simulink model "PStest"  (R2018a)
settings: Solver=VariableStepAuto  StartTime=0.0  StopTime=5  RelTol=1e-8
PreLoadFcn:
  | Ts_Power=50e-6;
  | Ts_Control=100e-6;
StopFcn:
  | clear C
  | C(1,:)={'Iterac',saveIte(1,1),saveIte(1,2),saveIte(1,3),saveIte(1,4)};
  | C(2,:)={'Time (sec)',saveIte(2,1),saveIte(2,2),saveIte(2,3),saveIte(2,4)};
  | C(3,:)={'Pmax',saveIte(3,1),saveIte(3,2),saveIte(3,3),saveIte(3,4)};
  | C(4,:)={'Duty',saveIte(4,1),saveIte(4,2),saveIte(4,3),saveIte(4,4)};
  | C(5,:)={'When',saveIte(5,1)*0.1,saveIte(5,2)*0.1,saveIte(5,3)*0.1,saveIte(5,4)*0.1};
  | C(6,:)={'Tolerac',saveIte(6,1),saveIte(6,2),saveIte(6,3),saveIte(6,4)};
  | openvar('C')
libraries: powerlib x19, re_lib x6, simulink x1
Description:
  | Copyright 2008-2018 The MathWorks, Inc.
settings Model: NumberOfSteps=8002  Creator=MathWorks  LastModifiedBy=Mortuus
settings DataIOCC: LimitDataPoints=on  SaveFormat=Array  SignalLoggingSaveFormat=ModelDataLogs
settings OptimizationCC: ExpressionDepthLimit=2147483647  LifeSpan=inf
settings DebuggingCC: AlgebraicLoopMsg=none  UnderspecifiedInitializationDetection=Classic  MergeDetectMultiDrivingBlocksExec=none  SolverPrmCheckMsg=warning  FcnCallInpInsideContextMsg=warning  StateNameClashWarn=warning  SFUnexpectedBacktrackingDiag=warning  SFNoUnconditionalDefaultTransitionDiag=warning  SFExecutionAtInitializationDiag=none
settings HardwareCC: ProdBitPerPointer=32  ProdBitPerSizeT=32  ProdBitPerPtrDiffT=32  ProdLargestAtomicFloat=None  ProdIntDivRoundTo=Undefined  ProdEndianess=Unspecified  ProdWordSize=32  ProdHWDeviceType=32-bit Generic
settings ModelReferenceCC: PropagateSignalLabelsOutOfModel=off
settings CodeAppCC: StateflowObjectComments=on
settings GRTTargetCC: TargetLangStandard=C89/C90 (ANSI)  GeneratePreprocessorConditionals=Disable all  CombineOutputUpdateFcns=off  GRTInterface=on
settings ConfigComp: CovMetricSettings=dw  CovHtmlReporting=on  CovSaveCumulativeToWorkspaceVar=on  CovSaveSingleToWorkspaceVar=on  CovExternalEMLEnable=off  CovSFcnEnable=off
settings SimscapeCC: SimscapeNormalizeSystem=off

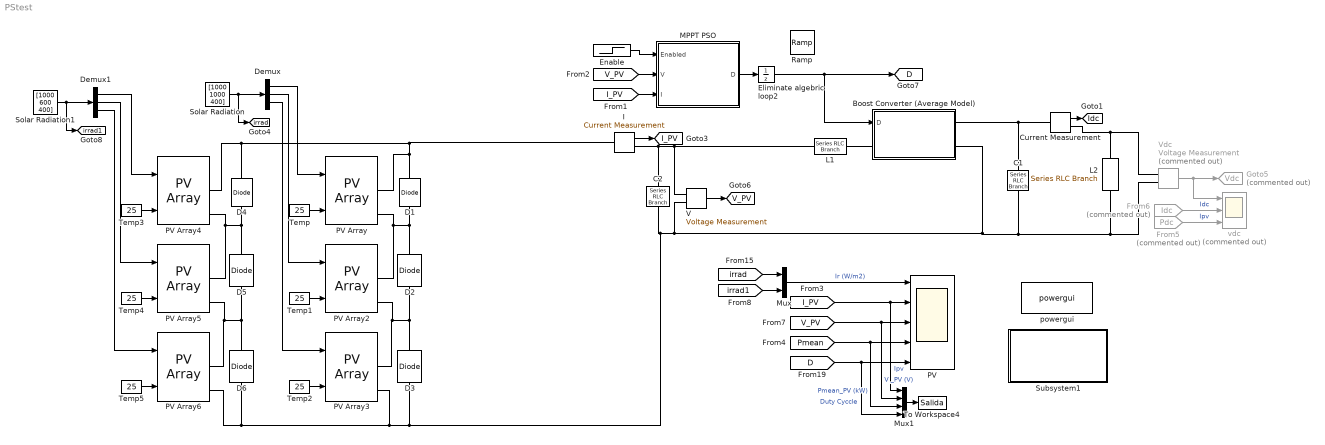
== system PStest ==
  Boost Converter (Average Model) : Subsystem  mask(Boost Converter (Average Model)){Ts=Ts_Power}
      mask prompts: Ts "Sample time:"
      mask Display: disp('Boost\n(Average)')
  C1 : powerlib/Elements/Series RLC Branch  LConnTagsString=__new0  RConnTagsString=__new0  BranchType=C  Resistance=1.0  Inductance=1.0  SetiL0=off  InitialCurrent=0  Capacitance=220e-06  Setx0=on  InitialVoltage=1  Measurements=None
  C2 : powerlib/Elements/Series RLC Branch  LConnTagsString=__new0  RConnTagsString=__new0  BranchType=C  Resistance=1.0  Inductance=1.0  SetiL0=off  InitialCurrent=0  Capacitance=470e-6  Setx0=on  InitialVoltage=50  Measurements=Branch voltage
  Current Measurement : powerlib/Measurements/Current Measurement  PhasorSimulation=off  OutputType=Magnitude  PSBequivalent=0
  D{1..6} (6 alike) : powerlib/Power Electronics/Diode  Ron=0.001  Lon=0  Vf=0.8  IC=0  UseSnubber=off  Rs=500  Cs=250e-9  Measurements=off
  Demux : Demux  Outputs=3
  Demux1 : Demux  Outputs=3
  Eliminate algebric loop2 : UnitDelay  SampleTime=Ts_Control
  Enable : Step  Time=0.01  SampleTime=0
  From5 : From  Commented=on  GotoTag=Pdc  TagVisibility=global
      settings: CloseFcn=tagdialog Close
  From6 : From  Commented=on  GotoTag=Idc  TagVisibility=global
      settings: CloseFcn=tagdialog Close
  Goto5 : Goto  Commented=on  GotoTag=Vdc  TagVisibility=global
  I : powerlib/Measurements/Current Measurement  PhasorSimulation=off  OutputType=Complex  PSBequivalent=0
  L1 : powerlib/Elements/Series RLC Branch  LConnTagsString=__new0  RConnTagsString=__new0  BranchType=RL  Resistance=0.3  Inductance=1e-3  SetiL0=off  InitialCurrent=0  Capacitance=1e-6  Setx0=off  InitialVoltage=0  Measurements=None
  L2 : powerlib/Elements/Series RLC Branch  LConnTagsString=__new0  RConnTagsString=__new0  BranchType=R  Resistance=100  Inductance=5e-3  SetiL0=off  InitialCurrent=0  Capacitance=1e-6  Setx0=off  InitialVoltage=0  Measurements=None
  "MPPT PSO " : MATLAB Function  TreatAsAtomicUnit=on  SystemSampleTime=0.1
  Mux : Mux  Inputs=2
  Mux1 : Mux
  PV : Scope  NumInputPorts=5
  PV Array{,2..6} (6 alike) : re_lib/Solar/PV Array  Npar=1  Nser=1  PlotType=array @ 25 deg.C & specified irradiances  S_vec="[ 1000  250 ]"  Temp_C_vec=[ 0 25 50]  ModuleName=User-defined  PlotWhenSelected=off  Pm=249.6159  Ncell=60  Voc=37.4  Isc=8.72  Vm=30.33  Im=8.23  beta_Voc_pc=-0.34  alpha_Isc_pc=0.07  beta_Voc=-0.12716  alpha_Isc=0.006104  IL=8.7463  I0=1.471e-10  nI=0.97837  Rsh=402.3586  Rs=0.31469  BAL=off  Tc=Tc  Tfilter=50e-6
  Ramp : simulink/Sources/Ramp  slope=-0.25  start=1  InitialOutput=1
  Solar Radiation : Constant  Value=[1000 1000 400]
  Solar Radiation1 : Constant  Value=[1000 600 400]
  Subsystem1 : Subsystem
      mask Display: disp('Additional \nscopes & measurements')
  Temp{,1..5} (6 alike) : Constant  Value=25
  To Workspace4 : ToWorkspace  VariableName=Salida  SaveFormat=Structure With Time  SampleTime=50e-6
      settings: Decimation=10
  V : powerlib/Measurements/Voltage Measurement  PhasorSimulation=off  OutputType=Complex  PSBequivalent=0
  "Vdc " : powerlib/Measurements/Voltage Measurement  Tag=PoWeRsYsTeMmEaSuReMeNt  Commented=on  PhasorSimulation=off  OutputType=Magnitude  PSBequivalent=0
  powergui : powerlib/powergui  Priority=1  SimulationMode=Continuous  SampleTime=Ts_Power  frequency=60  Iterations=50  frequencyindice=0  Pbase=100e6  ErrMax=1e-4  UnitsV=kV  UnitsW=MW  buscounter=0  FunctionMessages=off  echomessages=off  EnableUseOfTLC=off  CurrentSourceSwitches=off  DisableSnubberDevices=off  DisableRonSwitches=off  DisableVfSwitches=off  DisplayEquations=off  SolverType=Tustin/Backward Euler (TBE)  Interpol=off  ExternalGateDelay=off  methode=off  Ts=100  x0status=blocks  SPID=off  SwTol=0  HookPort=off  RestoreLinks=warning  ResistiveCurrentMeasurement=off  Frange=[0:2:500]  Ylog=off  Xlog=on  ShowGrid=off  save=off  variable=ZData  structure=0  ZoomFFT=on  StartTime=0.0  cycles=1  DisplayStyle=1  fundamental=60  FreqAxis=off  MaxFrequency=1000  frequencyindicesteady=1  RmsSteady=1  display=off
  vdc : Scope  Commented=on  NumInputPorts=3
  tag scope: D=global, I_PV=global, Idc=global, V_PV=global, irrad1=global, irrad=global
  wires:
  "MPPT PSO "/1(D) -> Eliminate algebric loop2/1
  [V_PV] -> "MPPT PSO "/2(V)
  [I_PV] -> "MPPT PSO "/3(I)
  Enable/1 -> "MPPT PSO "/1(Enabled)
  [Pmean] -> Mux1/3, PV/4  "Pmean_PV (kW)"
  [V_PV] -> Mux1/2, PV/3  "V _PV (V)"
  [I_PV] -> Mux1/1, PV/2  "Ipv"
  "Vdc "/1 -> vdc/1, Goto5/1
  Current Measurement/1 -> [Idc]
  From5/1 -> vdc/3  "Ipv"
  From6/1 -> vdc/2  "Idc"
  [D] -> Mux1/4, PV/5  "Duty Cyccle"
  I/1 -> [I_PV]
  V/1 -> [V_PV]
  Solar Radiation/1 -> [irrad], Demux/1
  Demux/1 -> PV Array/1
  Demux/2 -> PV Array2/1
  Demux/3 -> PV Array3/1
  Temp/1 -> PV Array/2
  Temp1/1 -> PV Array2/2
  Temp2/1 -> PV Array3/2
  Temp5/1 -> PV Array6/2
  Temp4/1 -> PV Array5/2
  Temp3/1 -> PV Array4/2
  Demux1/1 -> PV Array4/1
  Solar Radiation1/1 -> [irrad1], Demux1/1
  Demux1/3 -> PV Array6/1
  Demux1/2 -> PV Array5/1
  Eliminate algebric loop2/1 -> [D], Boost Converter (Average Model)/1(D)
  Mux/1 -> PV/1  "Ir (W/m2)"
  [irrad] -> Mux/1
  [irrad1] -> Mux/2
  Mux1/1 -> To Workspace4/1
  connections:
  L2/LConn1 -- Current Measurement/RConn1 -- "Vdc "/LConn1
  L1/RConn1 -- Boost Converter (Average Model)/LConn1
  Boost Converter (Average Model)/RConn1 -- Current Measurement/LConn1 -- C1/LConn1
  Boost Converter (Average Model)/RConn2 -- D6/LConn1 -- PV Array6/RConn2 -- PV Array3/RConn2 -- D3/LConn1 -- C2/RConn1 -- V/LConn2 -- C1/RConn1 -- L2/RConn1 -- "Vdc "/LConn2
  C2/LConn1 -- L1/LConn1 -- V/LConn1 -- I/RConn1
  D1/LConn1 -- D2/RConn1 -- PV Array2/RConn1 -- PV Array/RConn2
  D3/RConn1 -- PV Array2/RConn2 -- PV Array3/RConn1 -- D2/LConn1
  D1/RConn1 -- D4/RConn1 -- PV Array4/RConn1 -- I/LConn1 -- PV Array/RConn1
  PV Array6/RConn1 -- PV Array5/RConn2 -- D5/LConn1 -- D6/RConn1
  PV Array4/RConn2 -- PV Array5/RConn1 -- D5/RConn1 -- D4/LConn1

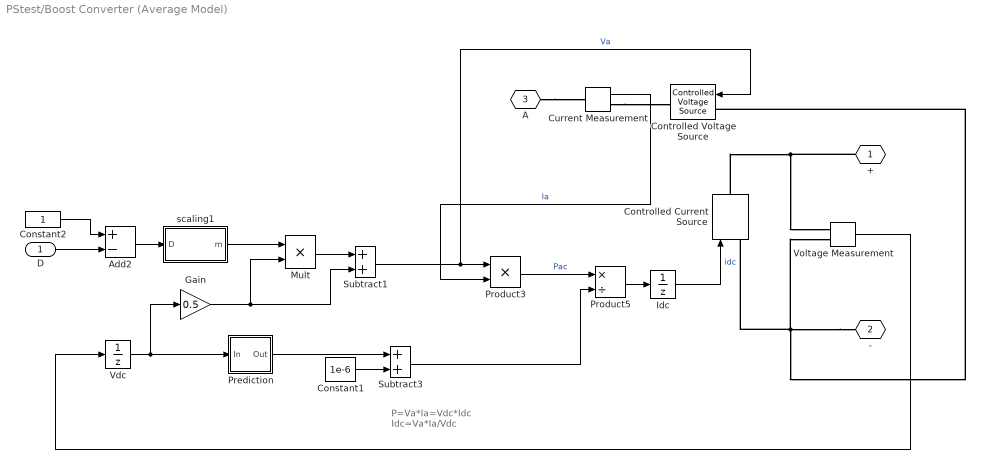
== system PStest/Boost Converter (Average Model) ==
  note: P=Va*Ia=Vdc*Idc
      | Idc=Va*Ia/Vdc
  D : Inport
  Add2 : Sum  Inputs=+-
  Constant1 : Constant  Value=1e-6
  Constant2 : Constant
  Controlled Current Source : powerlib/Electrical Sources/Controlled Current Source  Initialize=on  Source_Type=AC  Amplitude=0  Phase=0  Frequency=0  Measurements=None
  Controlled Voltage Source : powerlib/Electrical Sources/Controlled Voltage Source  Initialize=on  Source_Type=AC  Amplitude=0  Phase=0  Frequency=0  Measurements=None
  Current Measurement : powerlib/Measurements/Current Measurement  PhasorSimulation=off  OutputType=Complex  PSBequivalent=0
  Gain : Gain  Gain=0.5
  Idc : UnitDelay  SampleTime=Ts
  Mult : Product  Inputs=**
  Prediction : Subsystem
  Product3 : Product  RndMeth=Zero
  Product5 : Product  Inputs=*/  RndMeth=Zero
  Subtract1 : Sum
  Subtract3 : Sum
  Vdc : UnitDelay  SampleTime=Ts
  Voltage Measurement : powerlib/Measurements/Voltage Measurement  PhasorSimulation=off  OutputType=Complex  PSBequivalent=0
  scaling1 : Subsystem
  + : PMIOPort  Tag=PMCPort  Side=Right
  - : PMIOPort  Tag=PMCPort  Port=2  Side=Right
  A : PMIOPort  Tag=PMCPort  Port=3  Side=Left
  wires:
  Gain/1 -> Mult/2, Subtract1/2
  Product5/1 -> Idc/1
  Constant1/1 -> Subtract3/2
  Subtract3/1 -> Product5/2
  Product3/1 -> Product5/1  "Pac"
  Prediction/1(Out) -> Subtract3/1
  Vdc/1 -> Prediction/1(In), Gain/1
  Subtract1/1 -> Product3/1, Controlled Voltage Source/1  "Va"
  Mult/1 -> Subtract1/1
  Constant2/1 -> Add2/1
  Add2/1 -> scaling1/1(D)
  scaling1/1(m) -> Mult/1
  D/1 -> Add2/2
  Voltage Measurement/1 -> Vdc/1
  Idc/1 -> Controlled Current Source/1  "idc"
  Current Measurement/1 -> Product3/2  "Ia"
  connections:
  -/RConn1 -- Voltage Measurement/LConn2 -- Controlled Voltage Source/LConn1 -- Controlled Current Source/LConn1
  +/RConn1 -- Voltage Measurement/LConn1 -- Controlled Current Source/RConn1
  Current Measurement/RConn1 -- Controlled Voltage Source/RConn1
  A/RConn1 -- Current Measurement/LConn1

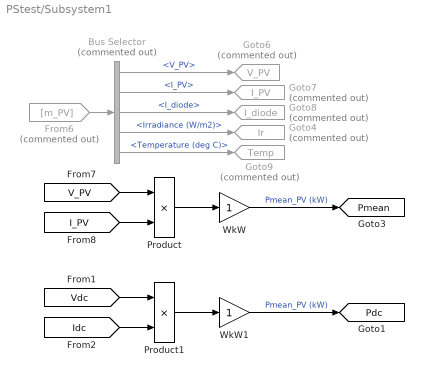
== system PStest/Subsystem1 ==
  Bus Selector : BusSelector  Commented=on  OutputSignals=V_PV,I_PV,I_diode,Irradiance (W/m2),Temperature (deg C)
  From6 : From  Commented=on  GotoTag=m_PV  TagVisibility=global
  Goto4 : Goto  Commented=on  GotoTag=Ir  TagVisibility=global
  Goto6 : Goto  Commented=on  GotoTag=V_PV  TagVisibility=global
  Goto7 : Goto  Commented=on  GotoTag=I_PV  TagVisibility=global
  Goto8 : Goto  Commented=on  GotoTag=I_diode  TagVisibility=global
  Goto9 : Goto  Commented=on  GotoTag=Temp  TagVisibility=global
  Product : Product  RndMeth=Zero
  Product1 : Product  RndMeth=Zero
  WkW : Gain
  WkW1 : Gain
  tag scope: Pdc=global, Pmean=global
  wires:
  [V_PV] -> Product/1
  Product/1 -> WkW/1
  [I_PV] -> Product/2
  Bus Selector/3 -> Goto8/1  "<I_diode>"
  Bus Selector/5 -> Goto9/1  "<Temperature (deg C)>"
  From6/1 -> Bus Selector/1
  Bus Selector/1 -> Goto6/1  "<V_PV>"
  Bus Selector/2 -> Goto7/1  "<I_PV>"
  Bus Selector/4 -> Goto4/1  "<Irradiance (W/m2)>"
  Product1/1 -> WkW1/1
  [Idc] -> Product1/2
  [Vdc] -> Product1/1
  WkW/1 -> [Pmean]  "Pmean_PV (kW)"
  WkW1/1 -> [Pdc]  "Pmean_PV (kW)"

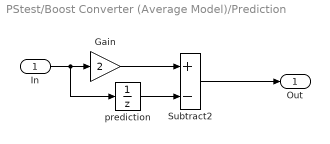
== system PStest/Boost Converter (Average Model)/Prediction ==
  In : Inport
  Gain : Gain  Gain=2
  Subtract2 : Sum  Inputs=+-
  prediction : UnitDelay  SampleTime=Ts
  Out : Outport
  wires:
  prediction/1 -> Subtract2/2
  In/1 -> prediction/1, Gain/1
  Subtract2/1 -> Out/1
  Gain/1 -> Subtract2/1

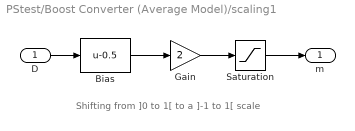
== system PStest/Boost Converter (Average Model)/scaling1 ==
  note: Shifting from ]0 to 1[ to a ]-1 to 1[ scale
  D : Inport
  Bias : Bias  Bias=-0.5
  Gain : Gain  Gain=2
  Saturation : Saturate  UpperLimit=1  LowerLimit=-1
  m : Outport
  wires:
  Saturation/1 -> m/1
  Gain/1 -> Saturation/1
  D/1 -> Bias/1
  Bias/1 -> Gain/1

== matlab function PStest/MPPT PSO  ==
  data: Enabled input; V input; I input; D output
function D = PandO(Enabled, V, I)
% coder.extrinsic('evaluar')
% [duty,P]=evaluar(20);
% MPPT controller based on the Perturb & Observe algorithm.
% D output = Duty cycle of the boost converter (value between 0 and 1)
% Enabled input = 1 to enable the MPPT controller
% V input = PV array terminal voltage (V)
% I input = PV array current (A)
% Param input:
Dinit = 0.5;  %Initial value for D output
Dmax = 0.9;   %Maximum value for D
Dmin = 0.2;   %Minimum value for D
deltaD = 0.01; %Increment value used to increase/decrease the duty cycle D
% ( increasing D = decreasing Vref )

persistent Vold Pold Dold;
dataType = 'double';
if isempty(Vold)
    Vold=0;
    Pold=0;
    Dold=Dinit;
end
P= V*I;
dV= V - Vold;
dP= P - Pold;
if dP ~= 0 & Enabled ~=0
    if dP < 0
        if dV < 0
            D = Dold - deltaD;
        else
            D = Dold + deltaD;
        end
    else
        if dV < 0
            D = Dold + deltaD;
        else
            D = Dold - deltaD;
        end    
    end
else D=Dold;
end
if D >= Dmax | D<= Dmin
    D=Dold;
end
Dold=D;
Vold=V;
Pold=P;
